simulink model "Matlab_Battery_Charge_RT"  (Simulink 8.5)
settings: Solver=ode3  SolverMode=SingleTasking  StartTime=0.0  StopTime=10  FixedStep=50e-6  RelTol=1e-3
undefined symbols (not defined in the file): another_event_name, Hydride, Metal, my_event_name, Nickel
libraries: powerlib x7, rtlab x2, artemis x1, electricdrivelib x1
settings Model: ARTEMISmethode_block_infos=$$__separator__$$Matlab_Battery_Charge_RT/ARTEMIS Guide$$__separator__$$  Creator=alsetlab  LastModifiedBy=alsetlab
settings DataIOCC: SignalLoggingSaveFormat=Dataset  SaveOutput=off  SaveTime=off
settings OptimizationCC: BlockReduction=off  OptimizeBlockIOStorage=off  BufferReuse=off  GlobalBufferReuse=off  ExpressionFolding=off  ExpressionDepthLimit=128  LocalBlockOutputs=off
settings DebuggingCC: UnderspecifiedInitializationDetection=Simplified  MergeDetectMultiDrivingBlocksExec=error  FcnCallInpInsideContextMsg=EnableAllAsError  StateNameClashWarn=none
settings GRTTargetCC: CombineOutputUpdateFcns=on  GRTInterface=off

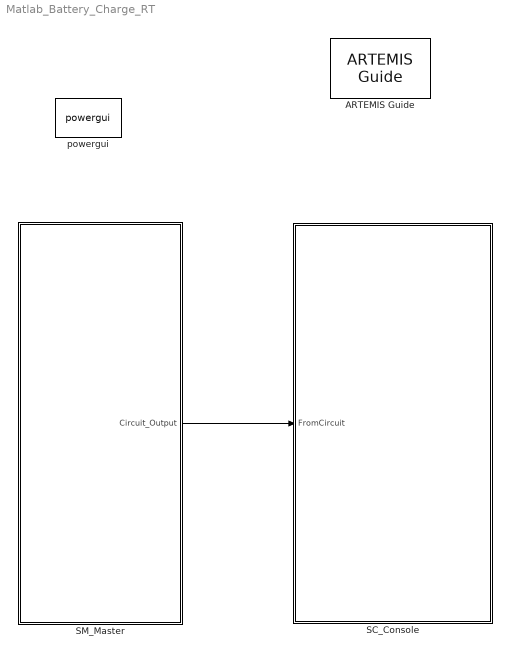
== system Matlab_Battery_Charge_RT ==
  ARTEMIS Guide : artemis/ARTEMIS/ARTEMIS Guide  Tag=FTSSmethode_opal_4hx0r99  Description=5.0_z1  lock=on  Ts=50e-6  opt=art5  dyna=off  nb_perm=4  RT_fullcomp=off  ssn=on  ssn_itvc=off  ssn_ivic=off  ssn_ext=off  ssn_solver=Art5  ssn_impulse=off  ssn_quasimpulse=off  ssn_impulse_loop=2  paraExtinctionThy=off  Thy_Impulse=on  dtc=Off  dtc_opt=normal  ao=on  simtype=off  ct_mac=off  lin_mov=off  lsp=[0.001 2]  spike_skip=Disabled  dtc_extra=1  dtc_sws=normal  dtc_pied=0.5  SPSRulesBlock=SPSRules  tre=on  ctmm=off  LF=off  dpl_type=ARTEMiS DPL  rlc_type=off  custom_type=off  para=on  ssn_ImpulseLoopBlockedStateUpdate=2  ssn_mov_iter_number=5  ssn_switch_iter_number=5  ssn_nib_type_verify=on  ssn_use_lu=on  ssn_use_ldlt=off
  SC_Console : Subsystem
  SM_Master : Subsystem
  powergui : powerlib/powergui  Priority=1  SimulationMode=Discrete  SolverType=Tustin  SampleTime=50e-6  frequency=60  SPID=off  DisableSnubberDevices=off  DisableRonSwitches=off  DisableVfSwitches=off  SwTol=0  DisplayEquations=off  Interpol=off  methode=off  Ts=100  FunctionMessages=off  echomessages=off  HookPort=off  EnableUseOfTLC=off  x0status=blocks  frequencyindice=0  Pbase=100e6  ErrMax=1e-4  Iterations=50  UnitsV=kV  UnitsW=MW  buscounter=0  RestoreLinks=warning  ResistiveCurrentMeasurement=off  Frange=[0:2:500]  Ylog=off  Xlog=on  ShowGrid=off  save=off  variable=ZData  structure=0  ZoomFFT=off  StartTime=0.0  cycles=1  DisplayStyle=1  fundamental=60  FreqAxis=off  MaxFrequency=1000  frequencyindicesteady=1  RmsSteady=1  display=off
  wires:
  SM_Master/1(Circuit_Output) -> SC_Console/1(FromCircuit)

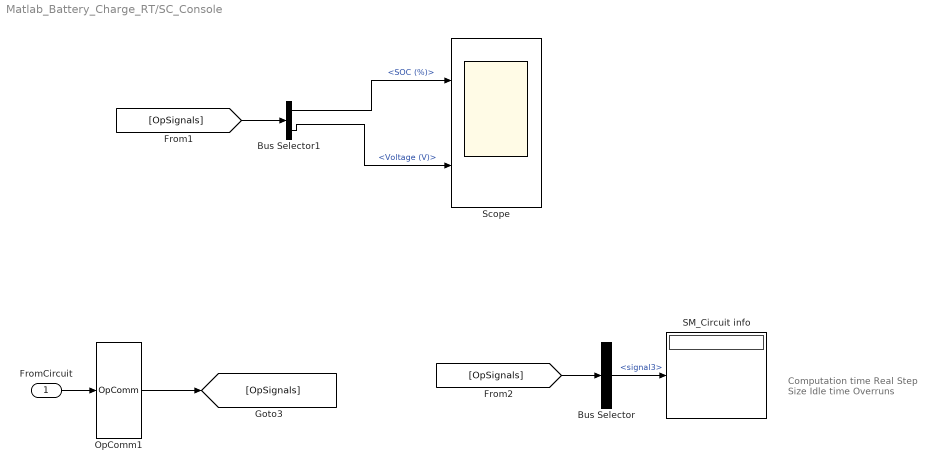
== system Matlab_Battery_Charge_RT/SC_Console ==
  note: Computation time
      | Real Step Size
      | Idle time
      | Overruns
  FromCircuit : Inport
  Bus Selector : BusSelector  OutputSignals=signal3
  Bus Selector1 : BusSelector  OutputSignals=SOC (%),Voltage (V)
  OpComm1 : rtlab/OpComm  nbport=1  groupe_acq=1  subsys_rate=0  st=0  Synchronization=on  Interpolation=on  Threshold=1  Missed_Data=off  Sim_Time=off  Samples=off  dynSigOut=off  from_console=0  warning_done=off  writeOpCommFile=off  Offset=off
  SM_Circuit info : Display
  Scope : Scope  NumInputPorts=2
      settings: YMin=-5~-5  YMax=5~5
  wires:
  Bus Selector/1 -> SM_Circuit info/1  "<signal3>"
  [OpSignals] -> Bus Selector/1
  OpComm1/1 -> [OpSignals]
  FromCircuit/1 -> OpComm1/1
  Bus Selector1/1 -> Scope/1  "<SOC (%)>"
  Bus Selector1/2 -> Scope/2  "<Voltage (V)>"
  [OpSignals] -> Bus Selector1/1

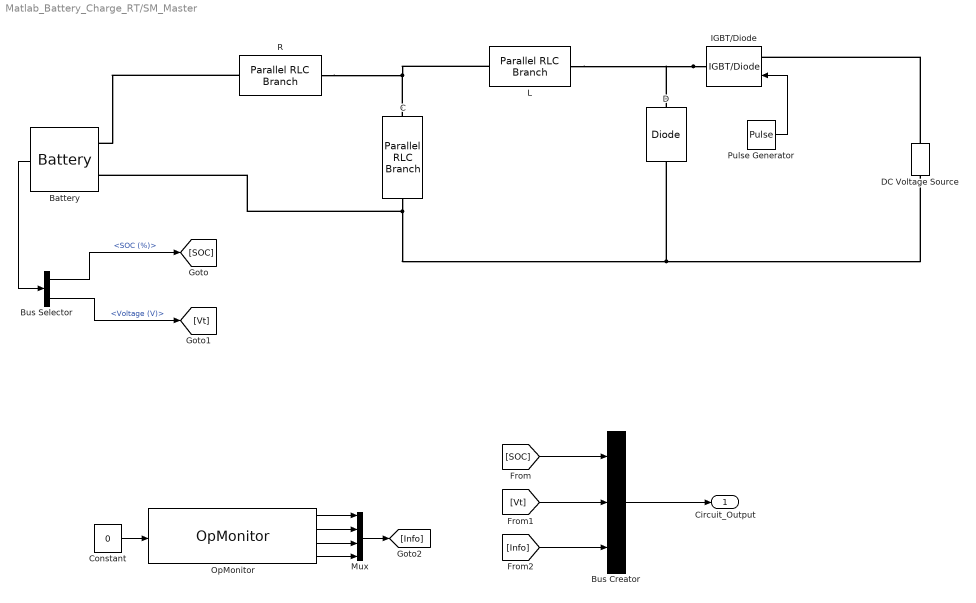
== system Matlab_Battery_Charge_RT/SM_Master ==
  Battery : electricdrivelib/Extra Sources/Battery  BatType=Nickel-Metal-Hydride  ShowDetailedParameters=off  NomV=3.5  NomQ=10  SOC=50  PresetModel=off  MaxQ=10.7692  FullV=4.1229  Dis_rate=2  R=0.005  Normal_OP=9.6154  expZone="[3.7966           2]"  current=[6.5 13 32.5]  Units=Time  Batt_Tr=30
  Bus Creator : BusCreator  Inputs=3
  Bus Selector : BusSelector  OutputSignals=SOC (%),Voltage (V)
  C : powerlib/Elements/Parallel RLC Branch  LConnTagsString=a  RConnTagsString=__new0  BranchType=C  Resistance=5  Inductance=1e-3  SetiL0=off  InitialCurrent=0  Capacitance=1000e-6  Setx0=off  InitialVoltage=0  Measurements=None
  Constant : Constant  Value=0
  D : powerlib/Power Electronics/Diode  Ron=0.01  Lon=0  Vf=0.8  IC=0  UseSnubber=off  Rs=500  Cs=250e-9  Measurements=off
  DC Voltage Source : powerlib/Electrical Sources/DC Voltage Source  Amplitude=8  Measurements=None
  IGBT/Diode : powerlib/Power Electronics/IGBT//Diode  Ron=1e-3  Rs=1e5  Cs=inf  Measurements=off
  L : powerlib/Elements/Parallel RLC Branch  LConnTagsString=a  RConnTagsString=__new0  BranchType=L  Resistance=1  Inductance=10e-3  SetiL0=off  InitialCurrent=0  Capacitance=1e-6  Setx0=off  InitialVoltage=0  Measurements=None
  Mux : Mux
  OpMonitor : rtlab/Monitoring/OpMonitor  compute_time=on  real_step=on  idle_time=on  nb_overruns=on  user_time=off  user_name=my_event_name,another_event_name
  Pulse Generator : DiscretePulseGenerator  PulseType=Time based  Period=0.002  PulseWidth=60
  R : powerlib/Elements/Parallel RLC Branch  LConnTagsString=a  RConnTagsString=__new0  BranchType=R  Resistance=0.005  Inductance=1e-3  SetiL0=off  InitialCurrent=0  Capacitance=1e-6  Setx0=off  InitialVoltage=0  Measurements=None
  Circuit_Output : Outport
  wires:
  Pulse Generator/1 -> IGBT/Diode/1
  Battery/1 -> Bus Selector/1
  Bus Selector/1 -> [SOC]  "<SOC (%)>"
  Bus Selector/2 -> [Vt]  "<Voltage (V)>"
  Bus Creator/1 -> Circuit_Output/1
  [Vt] -> Bus Creator/2
  Constant/1 -> OpMonitor/1
  Mux/1 -> [Info]
  OpMonitor/2 -> Mux/2
  OpMonitor/3 -> Mux/3
  OpMonitor/4 -> Mux/4
  OpMonitor/1 -> Mux/1
  [Info] -> Bus Creator/3
  [SOC] -> Bus Creator/1
  connections:
  C/LConn1 -- L/LConn1 -- R/LConn1
  IGBT/Diode/RConn1 -- L/RConn1 -- D/RConn1
  R/RConn1 -- Battery/LConn1
  C/RConn1 -- DC Voltage Source/LConn1 -- D/LConn1 -- Battery/LConn2
  DC Voltage Source/RConn1 -- IGBT/Diode/LConn1
